simulink model "msm_servo_loadest_dt"  (R2021b)
settings: Solver=VariableStepAuto  StartTime=0.0  StopTime=simlength  MaxStep=Tc  RelTol=Tc
values from neighbouring files (symbols this model uses):
  Aled = eye(4) + Ale*Ts    [msm_init.m]
  Bled = Ble*Ts    [msm_init.m]
  Cle = [1 0 0 0]    [msm_init.m]
  Kd = (K_hat+[1 0 0 0])/([C*Bd C*Ad; Bd Ad-eye(3)])    [msm_init.m]    (also in some_consideration.m = (K_hat+[0 0 0 1])/([Ad-eye(3) Bd; C*Ad C*Bd]))
  Lled = (dlqr(Aled',Cle',Q, R))'    [msm_init.m]
  load_torque = 10    [msm_init.m]
  simlength = 20    [msm_init.m]
  Tc = Ts    (= 0.0001)    [msm_init.m]
  Ts = 1/1e4    (= 0.0001)    [msm_init.m]
libraries: nesl_utility x5, fl_lib x4, mass_spring_mass_lib x1
settings Model: Creator=dbagn  LastModifiedBy=dbagn
settings SolverCC: AlgebraicLoopSolver=TrustRegion
settings DataIOCC: ReturnWorkspaceOutputs=off
settings DebuggingCC: SFMachineParentedDataDiag=warning

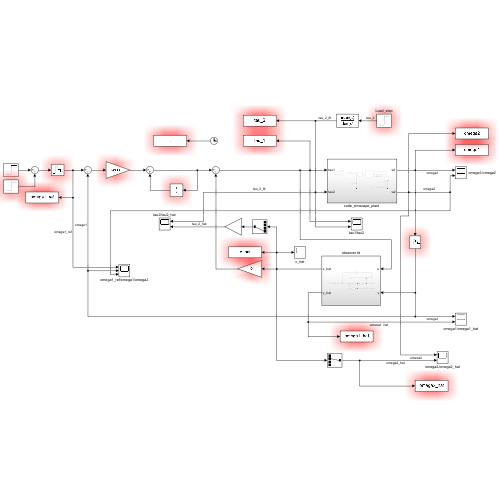
[thumbnail: Simulink's stored preview of the top-level diagram]
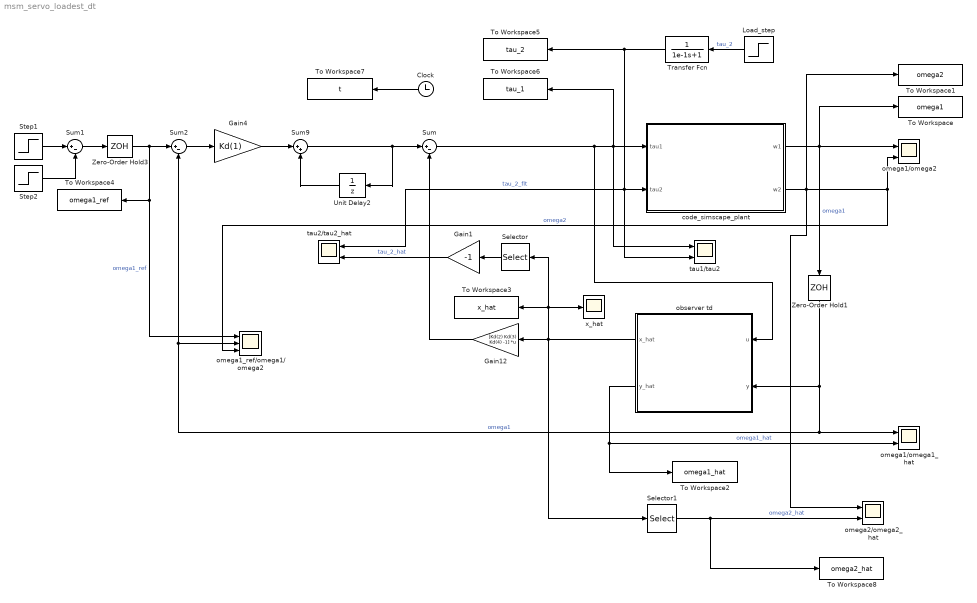
== system msm_servo_loadest_dt ==
  Clock : Clock
  Gain1 : Gain  Gain=-1
  Gain12 : Gain  Gain=[Kd(2) Kd(3) Kd(4) -1]  Multiplication=Matrix(K*u)
  Gain4 : Gain  Gain=Kd(1)
  Load_step : Step  Time=simlength/3  After=load_torque  SampleTime=0
  Selector : Selector  InputPortWidth=4  IndexOptions=Index vector (dialog)  Indices=4  OutputSizes=1
  Selector1 : Selector  InputPortWidth=4  IndexOptions=Index vector (dialog)  Indices=2  OutputSizes=1
  Step1 : Step  Time=0.2  SampleTime=0
  Step2 : Step  Time=simlength/2  SampleTime=0
  Sum : Sum  Inputs=|+-
  Sum1 : Sum  Inputs=|+-
  Sum2 : Sum  Inputs=|+-
  Sum9 : Sum  Inputs=|++
  To Workspace : ToWorkspace  VariableName=omega1  SampleTime=Tc
      settings: MaxDataPoints=Nc
  To Workspace1 : ToWorkspace  VariableName=omega2  SampleTime=Tc
      settings: MaxDataPoints=Nc
  To Workspace2 : ToWorkspace  VariableName=omega1_hat  SampleTime=Tc
      settings: MaxDataPoints=Nc
  To Workspace3 : ToWorkspace  VariableName=x_hat  SampleTime=Tc
      settings: MaxDataPoints=Nc
  To Workspace4 : ToWorkspace  VariableName=omega1_ref  SampleTime=Tc
      settings: MaxDataPoints=Nc
  To Workspace5 : ToWorkspace  VariableName=tau_2  SampleTime=Tc
      settings: MaxDataPoints=Nc
  To Workspace6 : ToWorkspace  VariableName=tau_1  SampleTime=Tc
      settings: MaxDataPoints=Nc
  To Workspace7 : ToWorkspace  VariableName=t  SampleTime=Tc
      settings: MaxDataPoints=Nc
  To Workspace8 : ToWorkspace  VariableName=omega2_hat  SampleTime=Tc
      settings: MaxDataPoints=Nc
  Transfer Fcn : TransferFcn  Denominator=[1e-1 1]
  Unit Delay2 : UnitDelay  SampleTime=Ts  HasFrameUpgradeWarning=on
  Zero-Order Hold1 : ZeroOrderHold  SampleTime=Ts
  Zero-Order Hold3 : ZeroOrderHold  SampleTime=Ts
  "code_simscape_plant " : Subsystem
  observer td : Subsystem
  omega1/omega1_hat : Scope  NumInputPorts=2
  omega1/omega2 : Scope  NumInputPorts=2
  omega1_ref/omega1/omega2 : Scope  NumInputPorts=3
  omega2/omega2_hat : Scope  NumInputPorts=2
  tau1/tau2 : Scope  NumInputPorts=2
  tau2/tau2_hat : Scope  NumInputPorts=2
  x_hat : Scope
  wires:
  "code_simscape_plant "/1(w1) -> Zero-Order Hold1/1, To Workspace/1, omega1/omega2/1  "omega1"
  "code_simscape_plant "/2(w2) -> To Workspace1/1, omega1/omega2/2, omega1_ref/omega1/omega2/3, omega2/omega2_hat/1  "omega2"
  observer td/2(y_hat) -> To Workspace2/1, omega1/omega1_hat/2  "omega1_hat"
  observer td/1(x_hat) -> Selector1/1, Selector/1, To Workspace3/1, x_hat/1, Gain12/1
  Gain4/1 -> Sum9/1
  Sum1/1 -> Zero-Order Hold3/1
  Zero-Order Hold3/1 -> To Workspace4/1, omega1_ref/omega1/omega2/1, Sum2/1  "omega1_ref"
  Load_step/1 -> Transfer Fcn/1  "tau_2"
  Zero-Order Hold1/1 -> omega1/omega1_hat/1, Sum2/2, omega1_ref/omega1/omega2/2, observer td/2(y)  "omega1"
  Gain12/1 -> Sum/2
  Clock/1 -> To Workspace7/1
  Sum2/1 -> Gain4/1
  Selector/1 -> Gain1/1
  Gain1/1 -> tau2/tau2_hat/2  "tau_2_hat"
  Selector1/1 -> To Workspace8/1, omega2/omega2_hat/2  "omega2_hat"
  Step1/1 -> Sum1/1
  Step2/1 -> Sum1/2
  Sum9/1 -> Sum/1, Unit Delay2/1
  Unit Delay2/1 -> Sum9/2
  Sum/1 -> tau1/tau2/1, "code_simscape_plant "/1(tau1), To Workspace6/1, observer td/1(u)
  Transfer Fcn/1 -> To Workspace5/1, tau1/tau2/2, tau2/tau2_hat/1, "code_simscape_plant "/2(tau2)  "tau_2_flt"

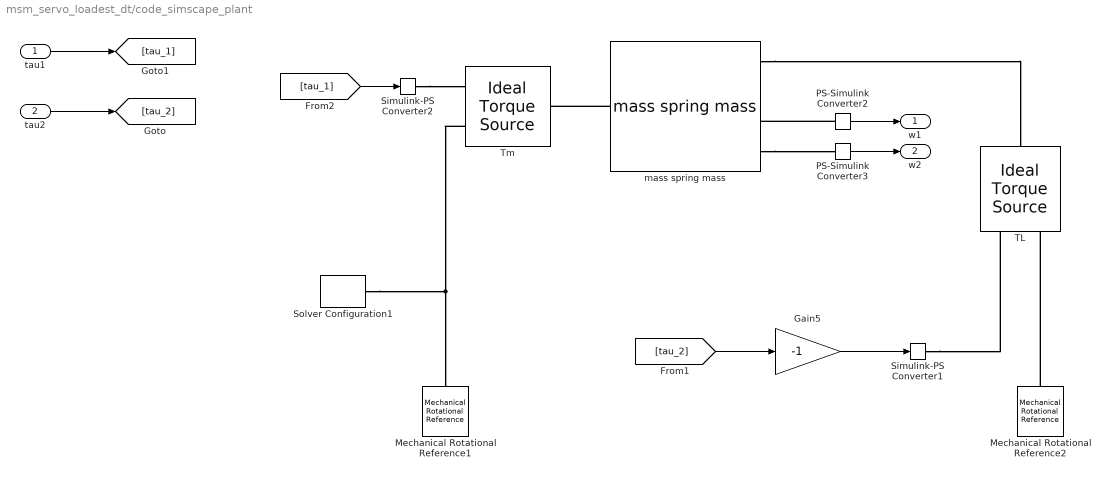
== system msm_servo_loadest_dt/code_simscape_plant  ==
  tau1 : Inport
  tau2 : Inport  Port=2
  Gain5 : Gain  Gain=-1
  Mechanical Rotational Reference1 : fl_lib/Mechanical/Rotational Elements/Mechanical Rotational Reference
  Mechanical Rotational Reference2 : fl_lib/Mechanical/Rotational Elements/Mechanical Rotational Reference
  PS-Simulink Converter2 : nesl_utility/PS-Simulink Converter  PhysicalDomain=network_engine_domain  SubClassName=ps_output  LeftPortType=input  RightPortType=output  PseudoPeriodic=off  Frequencies=[]  Unit=1  AffineConversion=off
      settings: SourceProductBaseCode=PW,SS
  PS-Simulink Converter3 : nesl_utility/PS-Simulink Converter  PhysicalDomain=network_engine_domain  SubClassName=ps_output  LeftPortType=input  RightPortType=output  PseudoPeriodic=off  Frequencies=[]  Unit=1  AffineConversion=off
      settings: SourceProductBaseCode=PW,SS
  Simulink-PS Converter1 : nesl_utility/Simulink-PS Converter  PhysicalDomain=network_engine_domain  SubClassName=ps_input  LeftPortType=input  RightPortType=output  PseudoPeriodic=off  Frequencies=[]  NoiseDistribution=none  NoiseParameters=[]  Unit=1  AffineConversion=off  FilteringAndDerivatives=provide  SimscapeFilterOrder=1  InputFilterTimeConstant=0.001  UdotUserProvided=0
      settings: SourceProductBaseCode=PW,SS
  Simulink-PS Converter2 : nesl_utility/Simulink-PS Converter  PhysicalDomain=network_engine_domain  SubClassName=ps_input  LeftPortType=input  RightPortType=output  PseudoPeriodic=off  Frequencies=[]  NoiseDistribution=none  NoiseParameters=[]  Unit=1  AffineConversion=off  FilteringAndDerivatives=provide  SimscapeFilterOrder=1  InputFilterTimeConstant=0.001  UdotUserProvided=0
      settings: SourceProductBaseCode=PW,SS
  Solver Configuration1 : nesl_utility/Solver Configuration  PhysicalDomain=network_engine_domain  SubClassName=solver  LeftPortType=input  RightPortType=generic  Tones=[]  Harmonics=[]  SimulateNoise=off  Profile=off  UseLocalSampling=off  EnableSwitchedLinearOptims=on  FrequencyDomain=off  UseCCode=off  RelTol=0.001  AbsTol=1e-06  MinStep=1e-09  ToWorkspace=off  RevertToSquareIcSolve=off  NumHomotopyIterations=100  PhasorMode=off  PhasorModeNumHarmonics=1  DoDC=off  ResidualTolerance=1e-09  UseLocalSolver=off  LocalSolverChoice=NE_TRAPEZOIDAL_ADVANCER  LocalSolverSampleTime=Tc  DoFixedCost=off  MaxNonlinIter=3  MaxModeIter=2  ComputeImpulses=off  ImpulseIterations=2  LinearAlgebra=auto  EquationFormulation=NE_TIME_EF  DelaysMemoryBudget=1024  AutomaticFiltering=on  FilteringTimeConstant=0.001  PartitionStorageMethod=AS_NEEDED  PartitionMemoryBudget=1024  PartitionMethod=ROBUST
      settings: SourceProductBaseCode=PW,SS
  TL : fl_lib/Mechanical/Mechanical Sources/Ideal Torque Source
  "Tm " : fl_lib/Mechanical/Mechanical Sources/Ideal Torque Source
  mass spring mass : mass_spring_mass_lib/mass spring mass  b1=b N*m/(rad/s)  J1=J1 kg*m^2  b2=b N*m/(rad/s)  J2=J2 kg*m^2  b_theta=b_theta N*m/(rad/s)  k_theta=k_theta N*m/rad  omega_1_specify=off  omega_1_priority=None  omega_1=0 rad/s  omega_1_nominal_specify=off  omega_1_nominal_unit=rad/s  omega_1_nominal_value=1  omega_2_specify=off  omega_2_priority=None  omega_2=0 rad/s  omega_2_nominal_specify=off  omega_2_nominal_unit=rad/s  omega_2_nominal_value=1  tau_1_specify=off  tau_1_priority=None  tau_1=0 N*m  tau_1_nominal_specify=off  tau_1_nominal_unit=N*m  tau_1_nominal_value=1  tau_2_specify=off  tau_2_priority=None  tau_2=0 N*m  tau_2_nominal_specify=off  tau_2_nominal_unit=N*m  tau_2_nominal_value=1  tau_theta_specify=off  tau_theta_priority=None  tau_theta=0 N*m  tau_theta_nominal_specify=off  tau_theta_nominal_unit=N*m  tau_theta_nominal_value=1
      settings: InternalSimscapePortConfiguration="{\"Bottom\":[],\"Left\":[{\"id\":\"S1\",\"label\":\"S1\",\"type\":\"foundation.mechanical.rotational.rotational\"}],\"Right\":[{\"id\":\"S2\",\"label\":\"S2\",\"type\":\"foundation.mechanical.rotational.rotational\"},{\"id\":\"tau_theta_out\",\"label\":\"tau_theta\",\"type\":\"output\"},{\"id\":\"omega1_out\",\"label\":\"omega1\",\"type\":\"output\"},{\"id\":\"omega2_out\",\"label\":\"omega2\",\"type\":\"output\"}],\"Top\":[]}"
  w1 : Outport
  w2 : Outport  Port=2
  wires:
  PS-Simulink Converter3/1 -> w2/1
  PS-Simulink Converter2/1 -> w1/1
  Gain5/1 -> Simulink-PS Converter1/1
  tau1/1 -> [tau_1]
  [tau_1] -> Simulink-PS Converter2/1
  tau2/1 -> [tau_2]
  [tau_2] -> Gain5/1
  connections:
  Simulink-PS Converter2/RConn1 -- "Tm "/RConn1
  mass spring mass/LConn1 -- "Tm "/LConn1
  Simulink-PS Converter1/RConn1 -- TL/RConn1
  mass spring mass/RConn1 -- TL/LConn1
  mass spring mass/RConn4 -- PS-Simulink Converter3/LConn1
  PS-Simulink Converter2/LConn1 -- mass spring mass/RConn3
  Solver Configuration1/RConn1 -- "Tm "/RConn2 -- Mechanical Rotational Reference1/LConn1
  Mechanical Rotational Reference2/LConn1 -- TL/RConn2

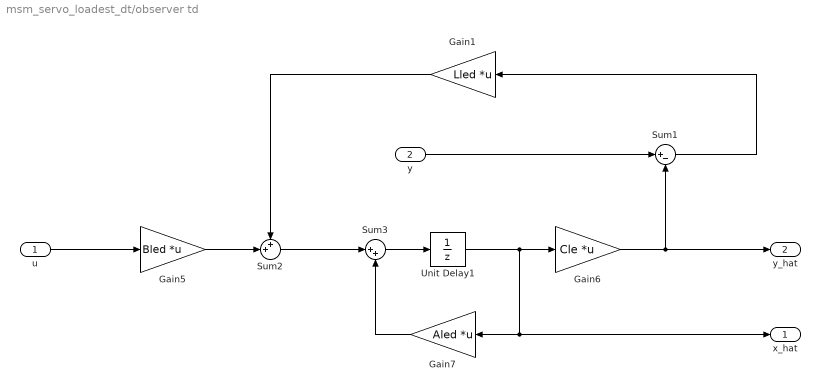
== system msm_servo_loadest_dt/observer td ==
  u : Inport
  y : Inport  Port=2
  Gain1 : Gain  Gain=Lled  Multiplication=Matrix(K*u)
  Gain5 : Gain  Gain=Bled  Multiplication=Matrix(K*u)
  Gain6 : Gain  Gain=Cle  Multiplication=Matrix(K*u)
  Gain7 : Gain  Gain=Aled  Multiplication=Matrix(K*u)
  Sum1 : Sum  Inputs=|+-
  Sum2 : Sum  Inputs=++|
  Sum3 : Sum  Inputs=|++
  Unit Delay1 : UnitDelay  SampleTime=Ts  HasFrameUpgradeWarning=on
  x_hat : Outport
  y_hat : Outport  Port=2
  wires:
  Sum2/1 -> Sum3/1
  Sum3/1 -> Unit Delay1/1
  Gain7/1 -> Sum3/2
  Gain6/1 -> y_hat/1, Sum1/2
  Sum1/1 -> Gain1/1
  u/1 -> Gain5/1
  Gain1/1 -> Sum2/1
  Gain5/1 -> Sum2/2
  Unit Delay1/1 -> x_hat/1, Gain7/1, Gain6/1
  y/1 -> Sum1/1
